simulink model "allActuatorCtrl_th"  (R2018b)
settings: Solver=VariableStepAuto  StartTime=0.0  StopTime=10.0  RelTol=1e-3
undefined symbols (not defined in the file or in its folder): eulerAngles, posVec, velocityVec
libraries: allActuatorCtrl_cl x1
settings Model: Creator=mcobb  LastModifiedBy=mcobb

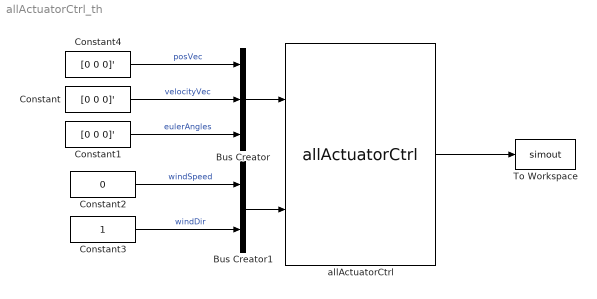
== system allActuatorCtrl_th ==
  Bus Creator : BusCreator  Inputs=posVec,velocityVec,eulerAngles  OutDataTypeStr=Bus: plantBus
  Bus Creator1 : BusCreator  Inputs=2  OutDataTypeStr=Bus: envBus  NonVirtualBus=on
      settings: InheritFromInputs=off
  Constant : Constant  Value=[0 0 0]'
  Constant1 : Constant  Value=[0 0 0]'
  Constant2 : Constant  Value=0
  Constant3 : Constant
  Constant4 : Constant  Value=[0 0 0]'
  To Workspace : ToWorkspace  VariableName=simout  SaveFormat=Timeseries  SampleTime=-1
  allActuatorCtrl : allActuatorCtrl_cl/allActuatorCtrl  SystemSampleTime=-1
  wires:
  Bus Creator/1 -> allActuatorCtrl/1
  Constant/1 -> Bus Creator/2  "velocityVec"
  Constant1/1 -> Bus Creator/3  "eulerAngles"
  Constant3/1 -> Bus Creator1/2  "windDir"
  Constant2/1 -> Bus Creator1/1  "windSpeed"
  Bus Creator1/1 -> allActuatorCtrl/2
  allActuatorCtrl/1 -> To Workspace/1
  Constant4/1 -> Bus Creator/1  "posVec"
